simulink model "volterra_sim"  (R2023b)
settings: Solver=VariableStepAuto  StartTime=0.0  StopTime=100  MaxStep=1e-4  RelTol=1e-3
settings Model: Creator=stefa  LastModifiedBy=stefa

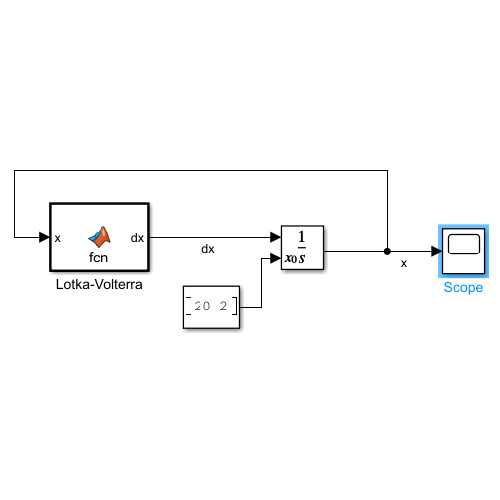
[thumbnail: Simulink's stored preview of the top-level diagram]
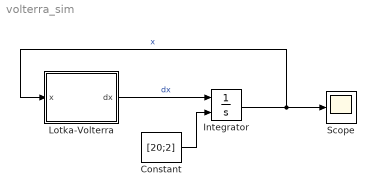
== system volterra_sim ==
  Constant : Constant  Value=[20;2]
  Integrator : Integrator  InitialConditionSource=external
  Lotka-Volterra : MATLAB Function  TreatAsAtomicUnit=on
  Scope : Scope
  wires:
  Lotka-Volterra/1(dx) -> Integrator/1  "dx"
  Constant/1 -> Integrator/2
  Integrator/1 -> Scope/1, Lotka-Volterra/1(x)  "x"

== matlab function volterra_sim/Lotka-Volterra ==
  data: x input; dx output
function dx = fcn(x)
x1=x(1);
x2=x(2);

a=1; %tasso natalità
b=0.5; %tasso che indica probabilità di incontro e capacità predatoria
gamma=1; %dinamica malthusiana
delta=0.5; % probabilità di incontro, capacità predatoria, conversione in biomassa

dx=[a*x1-b*x1*x2;
    -gamma*x2+delta*x1*x2];
